simulink model "firsttask"  (R2022a)
settings: Solver=VariableStepAuto  StartTime=0.0  StopTime=10.0  RelTol=1e-3
libraries: commdigbbndpm3 x4, simulink x4, commchan3 x2, commsink2 x2, commrandsrc3 x1
settings Model: Creator=Admin  LastModifiedBy=Admin
settings DataIOCC: LoadExternalInput=on

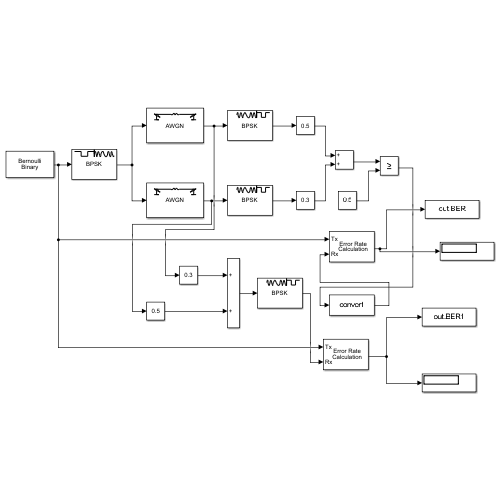
[thumbnail: Simulink's stored preview of the top-level diagram]
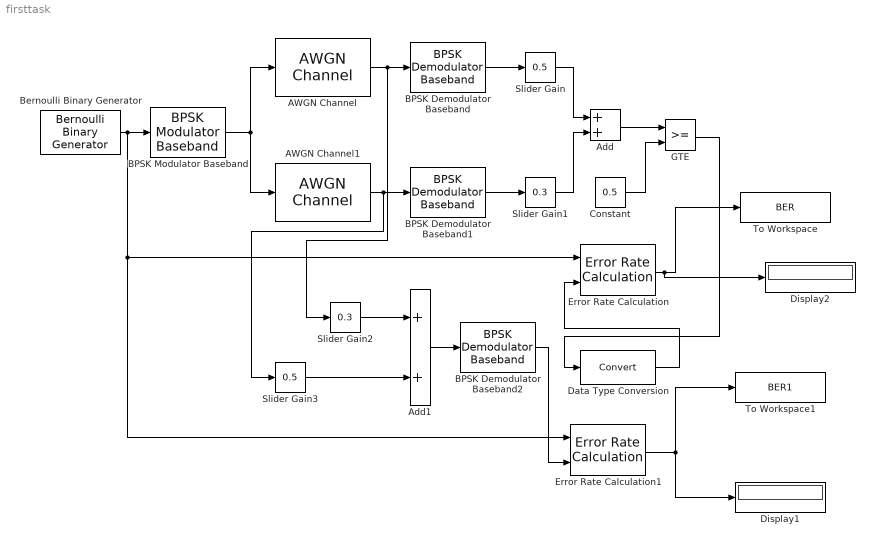
== system firsttask ==
  AWGN Channel : commchan3/AWGN Channel  InputProcessing=Columns as channels (frame based)  seed=67  noiseMode="Signal to noise ratio  (Eb/No)"  EbNodB=1  EsNodB=10  SNRdB=10  bitsPerSym=1  Ps=1  Tsym=1/1200  variance=1
  AWGN Channel1 : commchan3/AWGN Channel  InputProcessing=Columns as channels (frame based)  seed=67  noiseMode="Signal to noise ratio  (Eb/No)"  EbNodB=10  EsNodB=10  SNRdB=10  bitsPerSym=1  Ps=1  Tsym=1  variance=1
  Add : Sum
  Add1 : Sum
  BPSK Demodulator Baseband : commdigbbndpm3/BPSK Demodulator Baseband  DecType=Hard decision  VarSource=Dialog  Variance=1  Ph=0  outDtype=double  derotateFactorWordLen=16  derotateFactorDataTypeStr=Inherit: Same word length as input  derotateFactorLastDataTypeStr=Inherit: Same word length as input
  BPSK Demodulator Baseband1 : commdigbbndpm3/BPSK Demodulator Baseband  DecType=Hard decision  VarSource=Dialog  Variance=1  Ph=0  outDtype=double  derotateFactorWordLen=16  derotateFactorDataTypeStr=Inherit: Same word length as input  derotateFactorLastDataTypeStr=Inherit: Same word length as input
  BPSK Demodulator Baseband2 : commdigbbndpm3/BPSK Demodulator Baseband  DecType=Hard decision  VarSource=Dialog  Variance=1  Ph=0  outDtype=double  derotateFactorWordLen=16  derotateFactorDataTypeStr=Inherit: Same word length as input  derotateFactorLastDataTypeStr=Inherit: Same word length as input
  BPSK Modulator Baseband : commdigbbndpm3/BPSK Modulator Baseband  Ph=0  outDtype=double  outWordLen=16  outUDDataType=sfix(16)  outFracLenMode=Best precision  outFracLen=15  outDataTypeStr=double  outLastDataTypeStr=double
  Bernoulli Binary Generator : commrandsrc3/Bernoulli Binary Generator  ProbabilityOfZero=0.5  SeedSource=Auto  Seed=0  SampleTime=1/1200  SamplesPerFrame=1  OutputDataType=double  SimulateUsing=Interpreted execution
  Constant : Constant  Value=0.5
  Data Type Conversion : DataTypeConversion  SaturateOnIntegerOverflow=off  RndMeth=Floor
  Display1 : Display
  Display2 : Display
  Error Rate Calculation : commsink2/Error Rate Calculation  N=0  st_delay=0  cp_mode=Entire frame  subframe=[]  PMode=Port  WsName=ErrorVec  RsMode2=off  stop=off  numErr=100  maxBits=1e6
  Error Rate Calculation1 : commsink2/Error Rate Calculation  N=0  st_delay=0  cp_mode=Entire frame  subframe=[]  PMode=Port  WsName=ErrorVec  RsMode2=off  stop=off  numErr=100  maxBits=1e6
  GTE : RelationalOperator  OutDataTypeStr=boolean  RndMeth=Simplest  InputSameDT=off
  Slider Gain : simulink/Math Operations/Slider Gain  gain=0.5  low=0  high=2
  Slider Gain1 : simulink/Math Operations/Slider Gain  gain=0.3  low=0  high=2
  Slider Gain2 : simulink/Math Operations/Slider Gain  gain=0.3  low=0  high=2
  Slider Gain3 : simulink/Math Operations/Slider Gain  gain=0.5  low=0  high=2
  To Workspace : ToWorkspace  VariableName=BER  SaveFormat=Timeseries  SampleTime=-1
  To Workspace1 : ToWorkspace  VariableName=BER1  SaveFormat=Timeseries  SampleTime=-1
  wires:
  Bernoulli Binary Generator/1 -> Error Rate Calculation/1, Error Rate Calculation1/1, BPSK Modulator Baseband/1
  BPSK Modulator Baseband/1 -> AWGN Channel/1, AWGN Channel1/1
  AWGN Channel1/1 -> Slider Gain3/1, BPSK Demodulator Baseband1/1
  AWGN Channel/1 -> Slider Gain2/1, BPSK Demodulator Baseband/1
  BPSK Demodulator Baseband/1 -> Slider Gain/1
  BPSK Demodulator Baseband1/1 -> Slider Gain1/1
  Slider Gain1/1 -> Add/2
  Slider Gain/1 -> Add/1
  Add/1 -> GTE/1
  Constant/1 -> GTE/2
  Slider Gain3/1 -> Add1/2
  Slider Gain2/1 -> Add1/1
  Add1/1 -> BPSK Demodulator Baseband2/1
  BPSK Demodulator Baseband2/1 -> Error Rate Calculation1/2
  Data Type Conversion/1 -> Error Rate Calculation/2
  GTE/1 -> Data Type Conversion/1
  Error Rate Calculation/1 -> Display2/1, To Workspace/1
  Error Rate Calculation1/1 -> To Workspace1/1, Display1/1
